simulink model "full_wave_rectifification"  (R2024b)
settings: Solver=VariableStepAuto  StartTime=0.0  StopTime=10.0  MaxStep=1e-5  RelTol=1e-3
libraries: spsDiodeLib x4, spsACVoltageSourceLib x1, spsMeanLib x1, spsSeriesRLCBranchLib x1, spsVoltageMeasurementLib x1, sps_lib x1
settings Model: Creator=Admin  LastModifiedBy=pragy

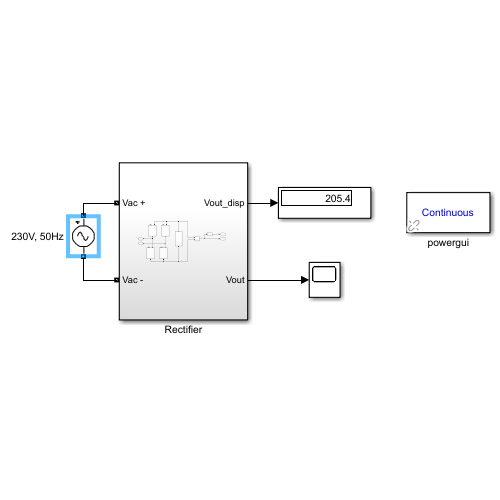
[thumbnail: Simulink's stored preview of the top-level diagram]
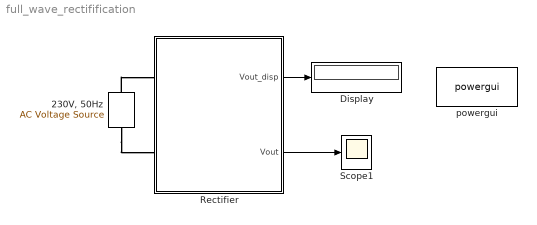
== system full_wave_rectifification ==
  "230V, 50Hz" : spsACVoltageSourceLib/AC Voltage Source  Amplitude=sqrt(2)*230  Phase=0  Frequency=50  SampleTime=0  Measurements=None  BusType=swing  Pref=10e3  Qref=0  Qmin=-inf  Qmax=+inf
  Display : Display
  Rectifier : Subsystem
  Scope1 : Scope
  powergui : sps_lib/powergui  Priority=1  SimulationMode=Continuous  SampleTime=50e-6  frequency=60  Iterations=50  frequencyindice=50  Pbase=100e6  ErrMax=1e-4  UnitsV=kV  UnitsW=MW  buscounter=0  FunctionMessages=off  echomessages=off  EnableUseOfTLC=off  CurrentSourceSwitches=off  DisableSnubberDevices=off  DisableRonSwitches=off  DisableVfSwitches=off  DisplayEquations=off  AutomaticDiscreteSolvers=off  SolverType=Tustin/Backward Euler (TBE)  Interpol=off  ExternalGateDelay=off  methode=off  Ts=100  x0status=zero  SPID=on  SwTol=0  HookPort=off  NonlinearTolerance=1e-4  nMaxIteration=100  ContinueOnMaxIteration=off  RestoreLinks=warning  ResistiveCurrentMeasurement=off  Frange=[0:2:500]  Ylog=off  Xlog=on  ShowGrid=off  save=off  variable=ZData  structure=0  ZoomFFT=off  StartTime=0.0  cycles=1  DisplayStyle=1  fundamental=60  FreqAxis=off  MaxFrequency=1000  frequencyindicesteady=1  RmsSteady=1  display=off
  wires:
  Rectifier/1(Vout_disp) -> Display/1
  Rectifier/2(Vout) -> Scope1/1
  connections:
  "230V, 50Hz"/RConn1 -- Rectifier/LConn1
  "230V, 50Hz"/LConn1 -- Rectifier/LConn2

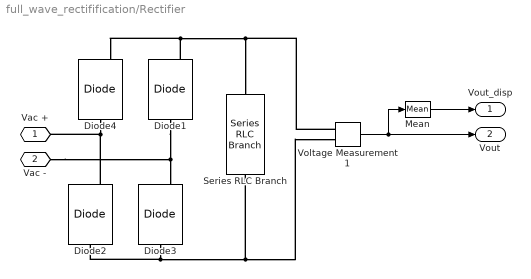
== system full_wave_rectifification/Rectifier ==
  Diode{1..4} (4 alike) : spsDiodeLib/Diode  Ron=0.001  Lon=0  Vf=0.8  IC=0  UseSnubber=0  Rs=500  Cs=250e-9  Measurements=on
  Mean : spsMeanLib/Mean  Freq=50  Vinit=0  Ts=0
  Series RLC Branch : spsSeriesRLCBranchLib/Series RLC Branch  LConnTagsString=__new0  RConnTagsString=__new0  BranchType=R  Resistance=10  Inductance=1000e-3  SetiL0=off  InitialCurrent=0  Capacitance=1e-6  Setx0=off  InitialVoltage=0  Measurements=None
  Voltage Measurement1 : spsVoltageMeasurementLib/Voltage Measurement  PhasorSimulation=off  OutputType=Complex  PSBequivalent=0
  Vac + : PMIOPort  Side=Left
  Vac - : PMIOPort  Port=2  Side=Left
  Vout_disp : Outport
  Vout : Outport  Port=2
  wires:
  Mean/1 -> Vout_disp/1
  Voltage Measurement1/1 -> Vout/1, Mean/1
  connections:
  Diode4/LConn1 -- Diode2/RConn1 -- Vac +/RConn1
  Diode1/RConn1 -- Series RLC Branch/LConn1 -- Voltage Measurement1/LConn1 -- Diode4/RConn1
  Diode1/LConn1 -- Vac -/RConn1 -- Diode3/RConn1
  Diode3/LConn1 -- Series RLC Branch/RConn1 -- Voltage Measurement1/LConn2 -- Diode2/LConn1
